simulink model "threedof"  (R2024a)
settings: Solver=VariableStepAuto  StartTime=0.0  StopTime=50  RelTol=1e-3
settings Model: Creator=rog  LastModifiedBy=rog

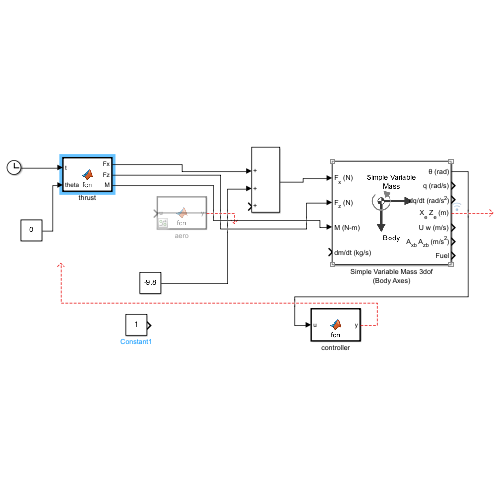
[thumbnail: Simulink's stored preview of the top-level diagram]
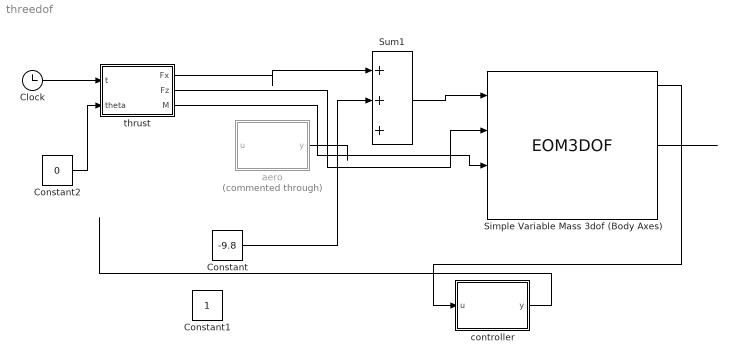
== system threedof ==
  Clock : Clock
  Constant : Constant  Value=-9.8
  Constant1 : Constant
  Constant2 : Constant  Value=0
  Simple Variable Mass 3dof (Body Axes) : EOM3DOF  mtype=Simple Variable  theta_ini=pi/2
  Sum1 : Sum  Inputs=|+++
  aero : MATLAB Function  Commented=through  TreatAsAtomicUnit=on
  controller : MATLAB Function  TreatAsAtomicUnit=on
  thrust : MATLAB Function  TreatAsAtomicUnit=on
  wires:
  aero/1(y) -> ?
  Clock/1 -> thrust/1(t)
  Constant2/1 -> thrust/2(theta)
  thrust/2(Fz) -> Simple Variable Mass 3dof (Body Axes)/2
  thrust/3(M) -> Simple Variable Mass 3dof (Body Axes)/3
  Constant/1 -> Sum1/2
  thrust/1(Fx) -> Sum1/1
  Sum1/1 -> Simple Variable Mass 3dof (Body Axes)/1
  Simple Variable Mass 3dof (Body Axes)/4 -> ?
  Simple Variable Mass 3dof (Body Axes)/1 -> controller/1(u)
  controller/1(y) -> ?

== matlab function threedof/controller ==
  data: u input; y output
function y = fcn(u)

y = u;

== matlab function threedof/thrust ==
  data: t input; Fx output; theta input; Fz output; M output
function [Fx, Fz, M]= fcn(t, theta)

if t < 5
    Fx = 50;
else
    Fx = 0;
end

Fz = 0;
M = 0;

== matlab function threedof/aero ==
  data: u input; y output
function y = fcn(u)

y = u;
